simulink model "A2_1_Elastisches_Getriebe_PR"  (R2023b)
settings: Solver=FixedStepAuto  StartTime=0.0  StopTime=10.0  FixedStep=1e-3  RelTol=1e-3
values from neighbouring files (symbols this model uses):
  A = [0 0 1 0; 0 0 0 1; 0 0.1e1 / CM / ig ^ 2 * c 0 0; 0 -(CM * ig ^ 2 + ms * s ^ 2 + CA) / CM / ig ^ 2 / (ms * s ^ 2 + CA) * c 0 0;]    [init_DSMS.m]    (also in init_DSMS_vorlage.m = [ 0 1 ; -c/m -d/m ]; init_elast_Getriebe.m = [0 0 1 0; 0 0 0 1; 0 0.1e1 / C_M_S / ig ^ 2 * c -0.1e1 / C_M; init_inverse_pendel_lin.m = [0 0 1 0; 0 0 0 1; 0 12 * m2 * s2 ^ 2 * g * l1 / (12 * (C_M_; init_inverse_pendel_pr.m = [0 0 0 1 0 0; 0 0 0 0 1 0; 0 0 0 0 0 1; 0 0.12e2 * l1 * g * )
  B = [0; 0; 0.1e1 / CM / ig; -0.1e1 / CM / ig;]    [init_DSMS.m]    (also in init_DSMS_vorlage.m = [ 0 1/m ]'; init_elast_Getriebe.m = [0; 0; 0.1e1 / C_M_S / ig; -0.1e1 / C_M_S / ig;]; init_inverse_pendel_lin.m = [0; 0; ig * (l2 ^ 2 + 12 * s2 ^ 2) / (12 * (C_M_S * ig ^ 2 +; init_inverse_pendel_pr.m = [0 0 0; 0 0 0; 0 0 0; 0.12e2 * ig * (((mP2 * l3 ^ 2 + m3 * s)
  C = diag([1, 1, 1, 1])    [init_DSMS.m]    (also in init_DSMS_vorlage.m = diag([1, 1]); init_elast_Getriebe.m = eye(4); init_inverse_pendel_lin.m = eye(4); init_inverse_pendel_pr.m = eye(6))
  D = zeros(size(C,1),size(B,2))    [init_DSMS.m]    (also in init_DSMS_vorlage.m; init_elast_Getriebe.m = [0; 0; 0; 0]; init_inverse_pendel_lin.m = [0; 0; 0; 0]; init_inverse_pendel_pr.m = [0 0 0; 0 0 0; 0 0 0; 0 0 0; 0 0 0; 0 0 0])
  k = lqr(sys, Q, R)    [init_elast_Getriebe.m]    (also in init_inverse_pendel_pr.m)
  V = 1/(-cT*inv(A-B*k)*B)    [init_elast_Getriebe.m]
  x1_ic = zeros(4,1)    [init_DSMS.m]    (also in init_DSMS_vorlage.m = zeros(2,1); init_elast_Getriebe.m; init_inv.m; init_inverse_pendel.m)
settings Model: Creator=Flo  LastModifiedBy=Flo

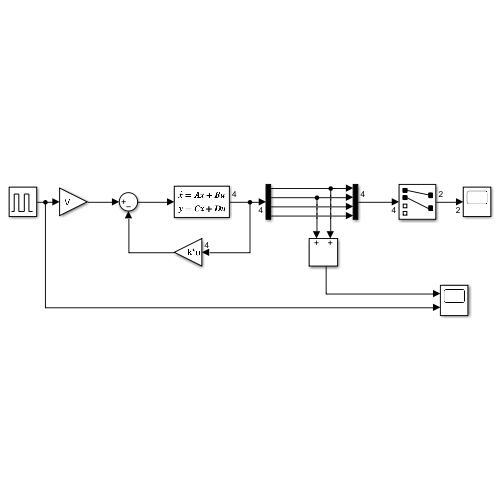
[thumbnail: Simulink's stored preview of the top-level diagram]
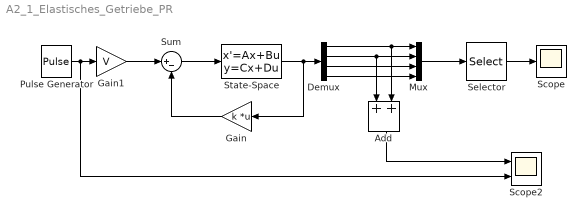
== system A2_1_Elastisches_Getriebe_PR ==
  Add : Sum
  Demux : Demux
  Gain : Gain  Gain=k  Multiplication=Matrix(K*u)
  Gain1 : Gain  Gain=V
  Mux : Mux
  Pulse Generator : DiscretePulseGenerator  PulseType=Time based  Period=5  PulseWidth=50
  Scope : Scope
  Scope2 : Scope  NumInputPorts=2
  Selector : Selector  InputPortWidth=4  IndexOptions=Index vector (dialog)  Indices=[1 2]  OutputSizes=1
  State-Space : StateSpace  A=A  B=B  C=C  D=D  InitialCondition=x1_ic
  Sum : Sum  Inputs=|+-
  wires:
  Selector/1 -> Scope/1
  Pulse Generator/1 -> Scope2/2, Gain1/1
  State-Space/1 -> Gain/1, Demux/1
  Demux/1 -> Mux/1, Add/2
  Demux/2 -> Mux/2, Add/1
  Demux/4 -> Mux/4
  Demux/3 -> Mux/3
  Mux/1 -> Selector/1
  Gain/1 -> Sum/2
  Sum/1 -> State-Space/1
  Add/1 -> Scope2/1
  Gain1/1 -> Sum/1
